simulink model "model"  (R2020a)
settings: Solver=FixedStepAuto  StartTime=0.0  StopTime=10.0  FixedStep=0.001  RelTol=1e-3  EnableMultiTasking=on
undefined symbols (not defined in the file or in its folder): para
settings Model: Creator=dddddx  LastModifiedBy=Administrator
settings DataIOCC: ReturnWorkspaceOutputs=off
settings OptimizationCC: LifeSpan=inf
settings DebuggingCC: SFUnexpectedBacktrackingDiag=warning  SFNoUnconditionalDefaultTransitionDiag=warning  ArithmeticOperatorsInVariantConditions=warning
settings SFSimCC: SimUseLocalCustomCode=off  CustomCodeUndefinedFunction=UseInterfaceOnly
settings RTWCC: RTWUseLocalCustomCode=off
settings CodeAppCC: StateflowObjectComments=on
settings GRTTargetCC: TargetLangStandard=C89/C90 (ANSI)
settings ConfigComp: CovMetricSettings=dw  CovHtmlReporting=on  CovSaveCumulativeToWorkspaceVar=on  CovSaveSingleToWorkspaceVar=on  CovExternalEMLEnable=off

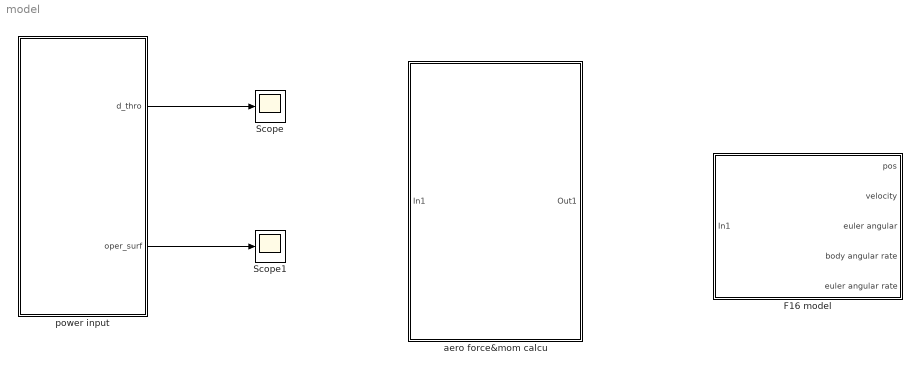
== system model ==
  "F16 model " : Subsystem
  Scope : Scope
  Scope1 : Scope
  aero force&mom calcu : Subsystem
  "power input " : Subsystem
  wires:
  "power input "/1(d_thro) -> Scope/1
  "power input "/2(oper_surf) -> Scope1/1

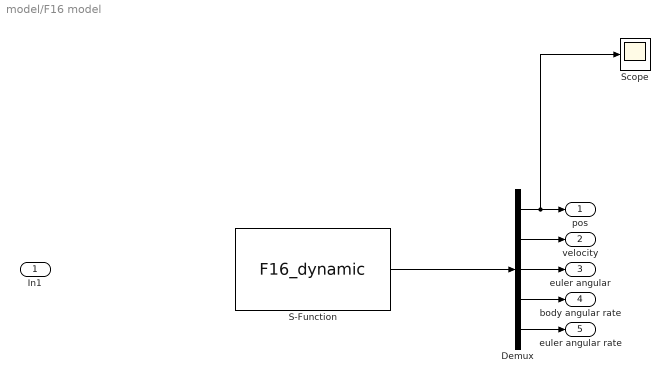
== system model/F16 model  ==
  In1 : Inport
  Demux : Demux  Outputs=5
  S-Function : S-Function  FunctionName=F16_dynamic  Parameters=para  SFunctionDeploymentMode=off  EnableBusSupport=off
  Scope : Scope
  pos : Outport  PortDimensions=3
  velocity : Outport  Port=2  PortDimensions=3
  euler angular : Outport  Port=3  PortDimensions=3
  body angular rate : Outport  Port=4  PortDimensions=3
  "euler angular rate " : Outport  Port=5  PortDimensions=3
  wires:
  Demux/4 -> body angular rate/1
  Demux/1 -> Scope/1, pos/1
  Demux/2 -> velocity/1
  S-Function/1 -> Demux/1
  Demux/3 -> euler angular/1
  Demux/5 -> "euler angular rate "/1

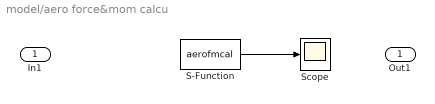
== system model/aero force&mom calcu ==
  In1 : Inport
  S-Function : S-Function  FunctionName=aerofmcal  Parameters=para  SFunctionDeploymentMode=off  EnableBusSupport=off
  Scope : Scope
  Out1 : Outport
  wires:
  S-Function/1 -> Scope/1

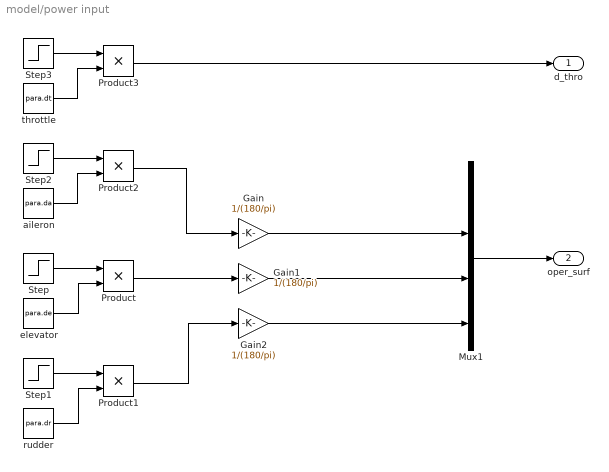
== system model/power input  ==
  " aileron" : Constant  Value=para.da
  Gain : Gain  Gain=1/(180/pi)
  Gain1 : Gain  Gain=1/(180/pi)
  Gain2 : Gain  Gain=1/(180/pi)
  Mux1 : Mux
  Product{,1..3} (4 alike) : Product
  Step{,1..3} (4 alike) : Step  Time=0  SampleTime=0
  elevator : Constant  Value=para.de
  rudder : Constant  Value=para.dr
  throttle : Constant  Value=para.dt  VectorParams1D=off
  d_thro : Outport
  oper_surf : Outport  Port=2
  wires:
  Step/1 -> Product/1
  elevator/1 -> Product/2
  Product/1 -> Gain1/1
  rudder/1 -> Product1/2
  Step1/1 -> Product1/1
  Product1/1 -> Gain2/1
  Step2/1 -> Product2/1
  Product2/1 -> Gain/1
  " aileron"/1 -> Product2/2
  Gain/1 -> Mux1/2
  Gain1/1 -> Mux1/3
  Gain2/1 -> Mux1/4
  Mux1/1 -> oper_surf/1
  Step3/1 -> Product3/1
  throttle/1 -> Product3/2
  Product3/1 -> d_thro/1
